simulink model "TRMSStateChart"  (R2020b)
settings: Solver=VariableStepAuto  StartTime=0.0  StopTime=inf  RelTol=1e-3
libraries: simulink x2
settings Model: EnablePacing=on  Creator=Ahmed Zaghloul  LastModifiedBy=Ahmed Zaghloul

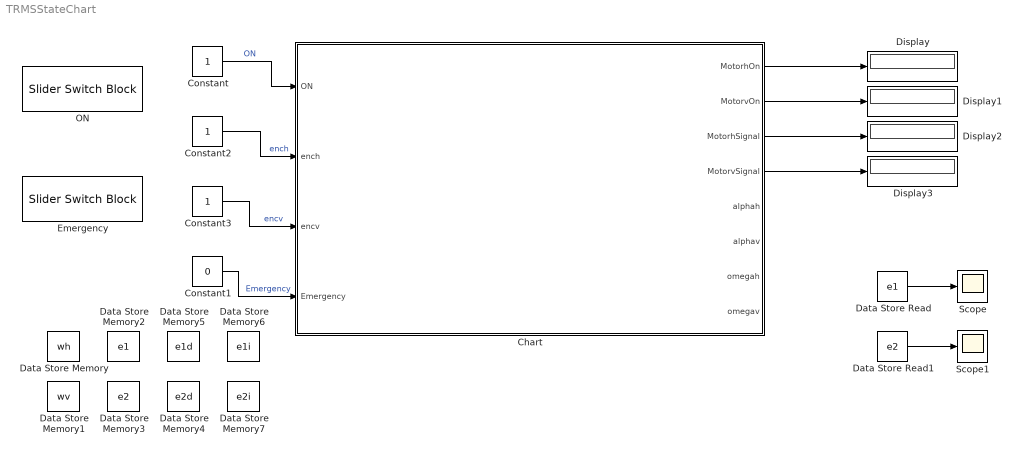
== system TRMSStateChart ==
  Chart : Stateflow chart  TreatAsAtomicUnit=on
  Constant : Constant
  Constant1 : Constant  Value=0
  Constant2 : Constant
  Constant3 : Constant
  Data Store Read : DataStoreRead  DataStoreName=e1
  Data Store Read1 : DataStoreRead  DataStoreName=e2
  Data Store Memory : DataStoreMemory  DataStoreName=wh  ReadBeforeWriteMsg=warning  WriteAfterWriteMsg=warning  WriteAfterReadMsg=warning  ShowAdditionalParam=off  OutDataTypeStr=double
  Data Store Memory1 : DataStoreMemory  DataStoreName=wv  ReadBeforeWriteMsg=warning  WriteAfterWriteMsg=warning  WriteAfterReadMsg=warning  ShowAdditionalParam=off  OutDataTypeStr=double
  Data Store Memory2 : DataStoreMemory  DataStoreName=e1  ReadBeforeWriteMsg=warning  WriteAfterWriteMsg=warning  WriteAfterReadMsg=warning  ShowAdditionalParam=off  OutDataTypeStr=double
  Data Store Memory3 : DataStoreMemory  DataStoreName=e2  ReadBeforeWriteMsg=warning  WriteAfterWriteMsg=warning  WriteAfterReadMsg=warning  ShowAdditionalParam=off  OutDataTypeStr=double
  Data Store Memory4 : DataStoreMemory  DataStoreName=e2d  ReadBeforeWriteMsg=warning  WriteAfterWriteMsg=warning  WriteAfterReadMsg=warning  ShowAdditionalParam=off  OutDataTypeStr=double
  Data Store Memory5 : DataStoreMemory  DataStoreName=e1d  ReadBeforeWriteMsg=warning  WriteAfterWriteMsg=warning  WriteAfterReadMsg=warning  ShowAdditionalParam=off  OutDataTypeStr=double
  Data Store Memory6 : DataStoreMemory  DataStoreName=e1i  ReadBeforeWriteMsg=warning  WriteAfterWriteMsg=warning  WriteAfterReadMsg=warning  ShowAdditionalParam=off  OutDataTypeStr=double
  Data Store Memory7 : DataStoreMemory  DataStoreName=e2i  ReadBeforeWriteMsg=warning  WriteAfterWriteMsg=warning  WriteAfterReadMsg=warning  ShowAdditionalParam=off  OutDataTypeStr=double
  Display{,1..3} (4 alike) : Display
  Emergency : SliderSwitchBlock
      settings: Values={{'Off', 'On'}, [0 1]}
  ON : SliderSwitchBlock
      settings: Values={{'Off', 'On'}, [0 1]}
  Scope : Scope
  Scope1 : Scope
  wires:
  Constant/1 -> Chart/1(ON)  "ON"
  Constant1/1 -> Chart/4(Emergency)  "Emergency"
  Chart/1(MotorhOn) -> Display/1
  Chart/2(MotorvOn) -> Display1/1
  Chart/3(MotorhSignal) -> Display2/1
  Chart/4(MotorvSignal) -> Display3/1
  Constant2/1 -> Chart/2(ench)  "ench"
  Constant3/1 -> Chart/3(encv)  "encv"
  Data Store Read/1 -> Scope/1
  Data Store Read1/1 -> Scope1/1

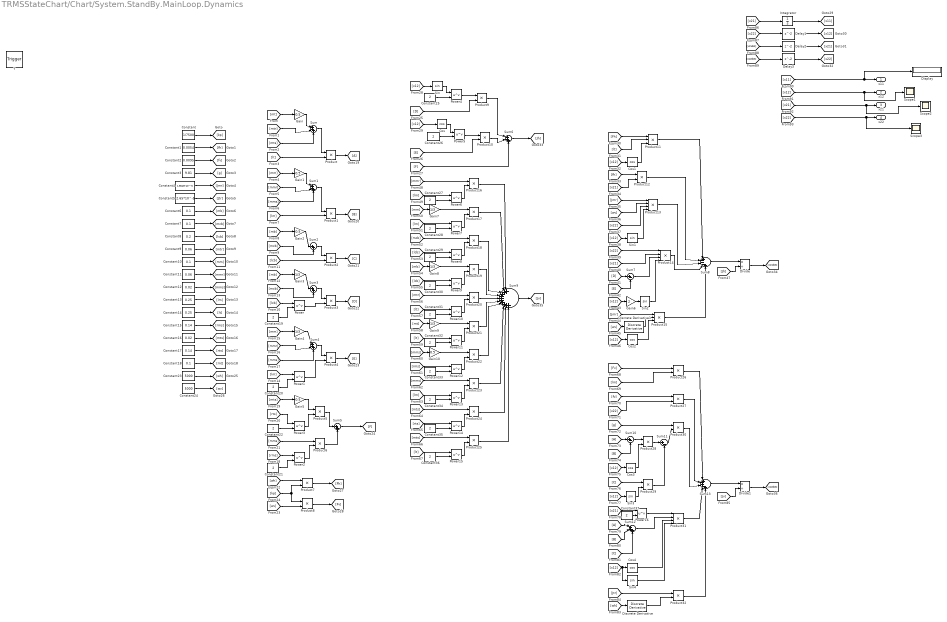
== system TRMSStateChart/Chart/System.StandBy.MainLoop.Dynamics ==
  f : TriggerPort  TriggerType=function-call  VariantControl=(inherit)  SampleTime=-1
      settings: CopyFcn=Stateflow.SLINSF.SimulinkMan.removeBlockPreDeleteFcn  PreDeleteFcn=Stateflow.SLINSF.SimulinkMan.unsafePredeleteFcn
  Constant : Constant  Value=1/7500
  Constant1 : Constant  Value=0.0054
  Constant{6..7,10,18} (4 alike) : Constant  Value=0.1
  Constant11 : Constant  Value=0.06
  Constant12 : Constant  Value=0.02
  Constant13 : Constant  Value=0.25
  Constant14 : Constant  Value=0.25
  Constant15 : Constant  Value=0.14
  Constant16 : Constant  Value=0.02
  Constant17 : Constant  Value=0.14
  Constant{19..22,25..37} (17 alike) : Constant  Value=2
  Constant2 : Constant  Value=0.0095
  Constant23 : Constant  Value=5000
  Constant24 : Constant  Value=5000
  Constant3 : Constant  Value=9.81
  Constant4 : Constant  Value=1.6543*10^-5
  Constant5 : Constant  Value=2.65*10^-5
  Constant8 : Constant  Value=0.2
  Constant9 : Constant  Value=0.06
  Cos{,1..4} (5 alike) : Trigonometry  Operator=cos
  Delay1 : Delay
  Delay2 : Delay
  Delay3 : Delay
  Discrete Derivative : simulink/Discrete/Discrete Derivative  gainval=1.0  ICPrevScaledInput=0.0  OutMin=[]  OutMax=[]  OutDataType=fixdt(1, 16)  OutScaling=2^-10  DoSatur=off
  Discrete Derivative1 : simulink/Discrete/Discrete Derivative  gainval=1.0  ICPrevScaledInput=0.0  OutMin=[]  OutMax=[]  OutDataType=fixdt(1, 16)  OutScaling=2^-10  DoSatur=off
  Display : Display
  Divide : Product  Inputs=*/
  Divide1 : Product  Inputs=*/
  Gain{,1..2,5,10} (5 alike) : Gain  Gain=0.5
  Gain{3..4,7..9} (5 alike) : Gain  Gain=1/3
  Gain6 : Gain  Gain=2
  Integrator : Integrator
  Power{,1..16} (17 alike) : Math  Operator=pow  SaturateOnIntegerOverflow=on
  Product{,1..10,12,16..30,32} (28 alike) : Product
  Product11 : Product  Inputs=3
  Product13 : Product  Inputs=4
  Product14 : Product  Inputs=4
  Product15 : Product  Inputs=3
  Product31 : Product  Inputs=4
  Scope1 : Scope
  Scope2 : Scope
  Scope3 : Scope
  Sin{,1..4} (5 alike) : Trigonometry
  Sum{,1,4,6,12} (5 alike) : Sum  Inputs=|+++
  Sum10 : Sum  Inputs=|+-
  Sum11 : Sum  Inputs=|+-
  Sum13 : Sum  Inputs=|+-+-+
  Sum2 : Sum  Inputs=|++
  Sum3 : Sum  Inputs=|++
  Sum5 : Sum  Inputs=|++
  Sum7 : Sum  Inputs=|+-
  Sum8 : Sum  Inputs=|+---+
  Sum9 : Sum  Inputs=|++++++++++
  x11 : Outport
  x12 : Outport  Port=2
  x21 : Outport  Port=3
  x22 : Outport  Port=4
  wires:
  Constant/1 -> [kp]
  Constant1/1 -> [fh]
  Constant2/1 -> [fv]
  Constant3/1 -> [g]
  Constant4/1 -> [Jmr]
  Constant5/1 -> [Jtr]
  Constant6/1 -> [mb]
  Constant7/1 -> [mcb]
  Constant8/1 -> [lcb]
  Constant9/1 -> [mtr]
  Constant10/1 -> [mm]
  Constant11/1 -> [mmr]
  Constant12/1 -> [mms]
  Constant13/1 -> [lm]
  Constant14/1 -> [lt]
  Constant15/1 -> [rms]
  Constant16/1 -> [mts]
  Constant17/1 -> [rts]
  [mt] -> Gain/1
  Constant18/1 -> [mt]
  Gain/1 -> Sum/1
  [mtr] -> Sum/2
  [mts] -> Sum/3
  [lt] -> Product/2
  Sum/1 -> Product/1
  Product/1 -> [A]
  Product1/1 -> [B]
  Sum1/1 -> Product1/1
  [lm] -> Product1/2
  [mms] -> Sum1/3
  [mmr] -> Sum1/2
  Gain1/1 -> Sum1/1
  [mm] -> Gain1/1
  Gain2/1 -> Sum2/1
  [lcb] -> Product2/2
  [mb] -> Gain2/1
  Product2/1 -> [C]
  [mcb] -> Sum2/2
  Sum2/1 -> Product2/1
  Sum3/1 -> Product3/1
  [mcb] -> Sum3/2
  Product3/1 -> [D]
  [mb] -> Gain3/1
  Gain3/1 -> Sum3/1
  [lcb] -> Power/1
  Constant19/1 -> Power/2
  Power/1 -> Product3/2
  Power1/1 -> Product4/2
  Constant20/1 -> Power1/2
  [lm] -> Power1/1
  Gain4/1 -> Sum4/1
  [mm] -> Gain4/1
  Product4/1 -> [E]
  [mmr] -> Sum4/2
  Sum4/1 -> Product4/1
  [mms] -> Sum4/3
  [rts] -> Power3/1
  Sum5/1 -> [F]
  [mts] -> Gain5/1
  Gain5/1 -> Product5/1
  [rms] -> Power2/1
  Constant21/1 -> Power2/2
  Constant22/1 -> Power3/2
  Power3/1 -> Product5/2
  Power2/1 -> Product6/2
  [mms] -> Product6/1
  Product5/1 -> Sum5/1
  Product6/1 -> Sum5/2
  Constant23/1 -> [wh]
  Constant24/1 -> [wv]
  [wh] -> Product7/1
  [kp] -> Product8/1, Product7/2
  [wv] -> Product8/2
  Product7/1 -> [Fh]
  Product8/1 -> [Fv]
  [x12] -> Sin/1
  Constant25/1 -> Power4/2
  Constant26/1 -> Power5/2
  Sin/1 -> Power4/1
  Power4/1 -> Product9/1
  [D] -> Product9/2
  [x12] -> Cos/1
  Cos/1 -> Power5/1
  Power5/1 -> Product10/1
  [E] -> Product10/2
  Product9/1 -> Sum6/1
  Product10/1 -> Sum6/2
  [F] -> Sum6/3
  Sum6/1 -> [Jh]
  [x12] -> Cos1/1
  [Fh] -> Product11/1
  [lt] -> Product11/2
  Cos1/1 -> Product11/3
  [fh] -> Product12/1
  [x21] -> Product12/2
  [x12] -> Sin1/1
  [Jmr] -> Product13/1
  [wv] -> Product13/2
  [x22] -> Product13/3
  Sin1/1 -> Product13/4
  [x12] -> Gain6/1
  Gain6/1 -> Sin2/1
  [x22] -> Product14/1
  [x21] -> Product14/2
  [D] -> Sum7/1
  [E] -> Sum7/2
  Sum7/1 -> Product14/3
  Sin2/1 -> Product14/4
  [x12] -> Cos2/1
  [Jmr] -> Product15/1
  Cos2/1 -> Product15/3
  Product11/1 -> Sum8/1
  Product12/1 -> Sum8/2
  Product13/1 -> Sum8/3
  Product14/1 -> Sum8/4
  Product15/1 -> Sum8/5
  Sum8/1 -> Divide/1
  [Jh] -> Divide/2
  Divide/1 -> [x21dot]
  [lm] -> Power6/1
  Constant27/1 -> Power6/2
  Power6/1 -> Product16/2
  [mmr] -> Product16/1
  [mm] -> Gain7/1
  Constant28/1 -> Power7/2
  [lm] -> Power7/1
  Gain7/1 -> Product17/1
  Power7/1 -> Product17/2
  [lcb] -> Power8/1
  Constant29/1 -> Power8/2
  [mcb] -> Product18/1
  Power8/1 -> Product18/2
  [mb] -> Gain8/1
  Constant30/1 -> Power9/2
  [lcb] -> Power9/1
  Gain8/1 -> Product19/1
  Power9/1 -> Product19/2
  Constant31/1 -> Power10/2
  [lt] -> Power10/1
  [mtr] -> Product20/1
  Power10/1 -> Product20/2
  [mt] -> Gain9/1
  Constant32/1 -> Power11/2
  [lt] -> Power11/1
  Gain9/1 -> Product21/1
  Power11/1 -> Product21/2
  [mms] -> Gain10/1
  Constant33/1 -> Power12/2
  [rms] -> Power12/1
  Gain10/1 -> Product22/1
  Power12/1 -> Product22/2
  Constant34/1 -> Power13/2
  [lm] -> Power13/1
  [mms] -> Product23/1
  Power13/1 -> Product23/2
  [lt] -> Power15/1
  [rts] -> Power14/1
  Constant36/1 -> Power15/2
  Constant35/1 -> Power14/2
  [mts] -> Product24/1
  Power14/1 -> Product24/2
  [mts] -> Product25/1
  Power15/1 -> Product25/2
  Product16/1 -> Sum9/1
  Product17/1 -> Sum9/2
  Product18/1 -> Sum9/3
  Product19/1 -> Sum9/4
  Product20/1 -> Sum9/5
  Product21/1 -> Sum9/6
  Product22/1 -> Sum9/7
  Product23/1 -> Sum9/8
  Product24/1 -> Sum9/9
  Product25/1 -> Sum9/10
  Sum9/1 -> [Jv]
  [Fv] -> Product26/1
  [lm] -> Product26/2
  [fv] -> Product27/1
  [x22] -> Product27/2
  [A] -> Sum10/1
  [B] -> Sum10/2
  [x12] -> Cos3/1
  Sum10/1 -> Product28/1
  Cos3/1 -> Product28/2
  [x12] -> Sin3/1
  Sin3/1 -> Product29/2
  [C] -> Product29/1
  Product28/1 -> Sum11/1
  Product29/1 -> Sum11/2
  [g] -> Product30/1
  Sum11/1 -> Product30/2
  Constant37/1 -> Power16/2
  [x21] -> Power16/1
  [A] -> Sum12/1
  [B] -> Sum12/2
  [C] -> Sum12/3
  [x12] -> Sin4/1, Cos4/1
  Power16/1 -> Product31/1
  Sum12/1 -> Product31/2
  Cos4/1 -> Product31/3
  Sin4/1 -> Product31/4
  [Jtr] -> Product32/1
  [wh] -> Discrete Derivative/1
  Product26/1 -> Sum13/1
  Product27/1 -> Sum13/2
  Product30/1 -> Sum13/3
  Product31/1 -> Sum13/4
  Product32/1 -> Sum13/5
  Sum13/1 -> Divide1/1
  [Jv] -> Divide1/2
  Divide1/1 -> [x22dot]
  Integrator/1 -> [x11]
  [x21] -> Integrator/1
  [x22] -> Delay1/1
  [x21dot] -> Delay2/1
  [x22dot] -> Delay3/1
  [x11] -> Display/1, x11/1
  [x12] -> Scope1/1, x12/1
  [x21] -> Scope2/1, x21/1
  [x22] -> Scope3/1, x22/1
  Delay1/1 -> [x12]
  Delay2/1 -> [x21]
  Delay3/1 -> [x22]
  Discrete Derivative/1 -> Product32/2
  [wv] -> Discrete Derivative1/1
  Discrete Derivative1/1 -> Product15/2

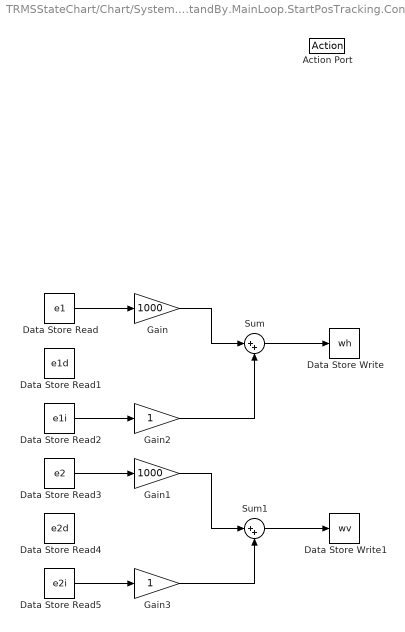
== system TRMSStateChart/Chart/System.StandBy.MainLoop.StartPosTracking.Controller ==
  Action Port : ActionPort
      settings: CopyFcn=Stateflow.SLINSF.SimulinkMan.removeBlockPreDeleteFcn  PreDeleteFcn=Stateflow.SLINSF.SimulinkMan.unsafePredeleteFcn
  Data Store Read : DataStoreRead  DataStoreName=e1
  Data Store Read1 : DataStoreRead  DataStoreName=e1d
  Data Store Read2 : DataStoreRead  DataStoreName=e1i
  Data Store Read3 : DataStoreRead  DataStoreName=e2
  Data Store Read4 : DataStoreRead  DataStoreName=e2d
  Data Store Read5 : DataStoreRead  DataStoreName=e2i
  Data Store Write : DataStoreWrite  DataStoreName=wh
  Data Store Write1 : DataStoreWrite  DataStoreName=wv
  Gain : Gain  Gain=1000
  Gain1 : Gain  Gain=1000
  Gain2 : Gain
  Gain3 : Gain
  Sum : Sum  Inputs=|++
  Sum1 : Sum  Inputs=|++
  wires:
  Data Store Read/1 -> Gain/1
  Data Store Read3/1 -> Gain1/1
  Data Store Read2/1 -> Gain2/1
  Data Store Read5/1 -> Gain3/1
  Gain/1 -> Sum/1
  Gain2/1 -> Sum/2
  Gain1/1 -> Sum1/1
  Gain3/1 -> Sum1/2
  Sum/1 -> Data Store Write/1
  Sum1/1 -> Data Store Write1/1

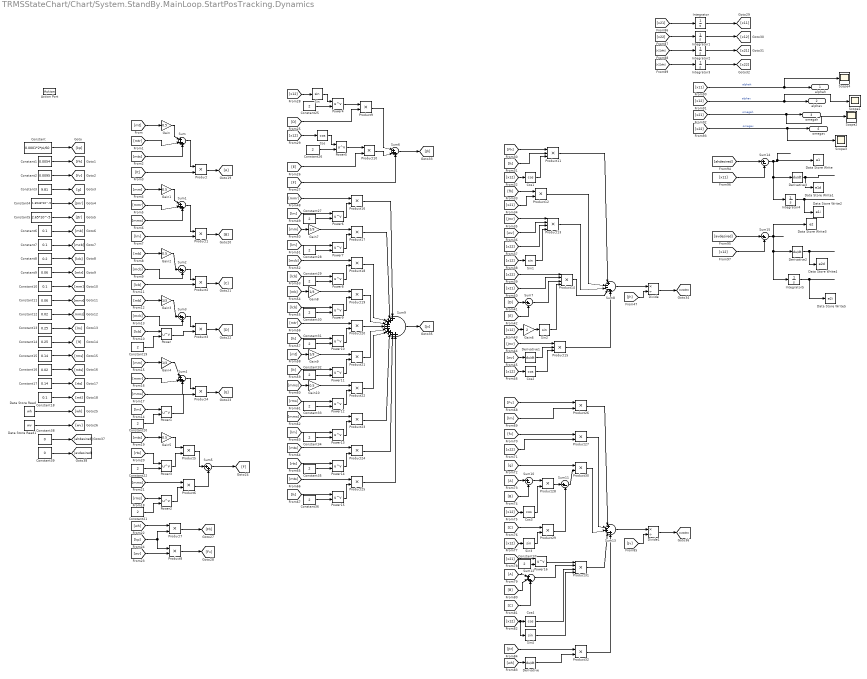
== system TRMSStateChart/Chart/System.StandBy.MainLoop.StartPosTracking.Dynamics ==
  Action Port : ActionPort
      settings: CopyFcn=Stateflow.SLINSF.SimulinkMan.removeBlockPreDeleteFcn  PreDeleteFcn=Stateflow.SLINSF.SimulinkMan.unsafePredeleteFcn
  Constant : Constant  Value=0.0001*2*pi/60
  Constant1 : Constant  Value=0.0054
  Constant{6..7,10,18} (4 alike) : Constant  Value=0.1
  Constant11 : Constant  Value=0.06
  Constant12 : Constant  Value=0.02
  Constant13 : Constant  Value=0.25
  Constant14 : Constant  Value=0.25
  Constant15 : Constant  Value=0.14
  Constant16 : Constant  Value=0.02
  Constant17 : Constant  Value=0.14
  Constant{19..22,25..37} (17 alike) : Constant  Value=2
  Constant2 : Constant  Value=0.0095
  Constant3 : Constant  Value=9.81
  Constant38 : Constant  Value=0
  Constant39 : Constant  Value=0
  Constant4 : Constant  Value=1.6543*10^-5
  Constant5 : Constant  Value=2.65*10^-5
  Constant8 : Constant  Value=0.2
  Constant9 : Constant  Value=0.06
  Cos{,1..4} (5 alike) : Trigonometry  Operator=cos
  Data Store Read : DataStoreRead  DataStoreName=wh
  Data Store Read1 : DataStoreRead  DataStoreName=wv
  Data Store Write : DataStoreWrite  DataStoreName=e1
  Data Store Write1 : DataStoreWrite  DataStoreName=e1d
  Data Store Write2 : DataStoreWrite  DataStoreName=e1i
  Data Store Write3 : DataStoreWrite  DataStoreName=e2
  Data Store Write4 : DataStoreWrite  DataStoreName=e2d
  Data Store Write5 : DataStoreWrite  DataStoreName=e2i
  Derivative{,1..3} (4 alike) : Derivative
  Divide : Product  Inputs=*/
  Divide1 : Product  Inputs=*/
  Gain{,1..2,5,10} (5 alike) : Gain  Gain=0.5
  Gain{3..4,7..9} (5 alike) : Gain  Gain=1/3
  Gain6 : Gain  Gain=2
  Integrator : Integrator  InitialCondition=0.1  WrapState=on  ContinuousStateAttributes='alphah'
  Integrator1 : Integrator  InitialCondition=0.1  WrapState=on  ContinuousStateAttributes='alphav'
  Integrator{2..5} (4 alike) : Integrator  ContinuousStateAttributes='omegah'
  Power{,1..16} (17 alike) : Math  Operator=pow  SaturateOnIntegerOverflow=on
  Product{,1..10,12,16..30,32} (28 alike) : Product
  Product11 : Product  Inputs=3
  Product13 : Product  Inputs=4
  Product14 : Product  Inputs=4
  Product15 : Product  Inputs=3
  Product31 : Product  Inputs=4
  Scope{1..4} (4 alike) : Scope
  Sin{,1..4} (5 alike) : Trigonometry
  Sum{,1,4,6,12} (5 alike) : Sum  Inputs=|+++
  Sum{7,10..11,14..15} (5 alike) : Sum  Inputs=|+-
  Sum13 : Sum  Inputs=|+-+-+
  Sum2 : Sum  Inputs=|++
  Sum3 : Sum  Inputs=|++
  Sum5 : Sum  Inputs=|++
  Sum8 : Sum  Inputs=|+---+
  Sum9 : Sum  Inputs=|++++++++++
  alphah : Outport
  alphav : Outport  Port=2
  omegah : Outport  Port=3
  omegav : Outport  Port=4
  wires:
  [x21] -> Integrator/1
  Constant3/1 -> [g]
  [mcb] -> Product18/1
  [F] -> Sum6/3
  [mm] -> Gain4/1
  Gain3/1 -> Sum3/1
  [C] -> Product29/1
  [fh] -> Product12/1
  [wh] -> Product7/1
  [x21] -> Power16/1
  [mb] -> Gain2/1
  Constant7/1 -> [mcb]
  [lm] -> Power6/1
  [x12] -> Sin4/1, Cos4/1
  Constant37/1 -> Power16/2
  Constant36/1 -> Power15/2
  [Jtr] -> Product32/1
  Product15/1 -> Sum8/5
  [rts] -> Power14/1
  Sin3/1 -> Product29/2
  Gain2/1 -> Sum2/1
  Constant5/1 -> [Jtr]
  [E] -> Product10/2
  Constant8/1 -> [lcb]
  Product2/1 -> [C]
  Gain10/1 -> Product22/1
  Product21/1 -> Sum9/6
  Sum10/1 -> Product28/1
  Product5/1 -> Sum5/1
  [x12] -> Cos3/1
  Constant21/1 -> Power2/2
  Sum/1 -> Product/1
  [lcb] -> Power9/1
  Sum9/1 -> [Jv]
  Product24/1 -> Sum9/9
  Product18/1 -> Sum9/3
  [x12] -> Cos/1
  Sum1/1 -> Product1/1
  [x22] -> Product27/2
  Divide/1 -> [x21dot]
  Constant34/1 -> Power13/2
  Power11/1 -> Product21/2
  [Jmr] -> Product15/1
  [mms] -> Product23/1
  Gain4/1 -> Sum4/1
  [wv] -> Product13/2
  Gain9/1 -> Product21/1
  [rms] -> Power12/1
  Power/1 -> Product3/2
  [mms] -> Gain10/1
  Constant33/1 -> Power12/2
  Constant28/1 -> Power7/2
  [mts] -> Product24/1
  [lt] -> Power15/1
  Gain8/1 -> Product19/1
  Power8/1 -> Product18/2
  [lt] -> Power11/1
  [lt] -> Power10/1
  Constant31/1 -> Power10/2
  Product7/1 -> [Fh]
  Constant35/1 -> Power14/2
  Constant32/1 -> Power11/2
  [mt] -> Gain/1
  Sum5/1 -> [F]
  [mtr] -> Product20/1
  Power9/1 -> Product19/2
  Constant30/1 -> Power9/2
  Sum8/1 -> Divide/1
  [Jh] -> Divide/2
  [lm] -> Power7/1
  Constant20/1 -> Power1/2
  [x21] -> Product14/2
  [mmr] -> Product16/1
  Constant27/1 -> Power6/2
  Gain7/1 -> Product17/1
  Product9/1 -> Sum6/1
  Product13/1 -> Sum8/3
  [lcb] -> Power8/1
  [x12] -> Cos2/1
  [mts] -> Gain5/1
  Cos2/1 -> Product15/3
  Power7/1 -> Product17/2
  Product1/1 -> [B]
  Cos/1 -> Power5/1
  [E] -> Sum7/2
  Product27/1 -> Sum13/2
  Sin2/1 -> Product14/4
  [x22] -> Product14/1
  Constant2/1 -> [fv]
  [x12] -> Gain6/1
  Sum11/1 -> Product30/2
  Constant15/1 -> [rms]
  Constant17/1 -> [rts]
  Gain6/1 -> Sin2/1
  Sum7/1 -> Product14/3
  Product6/1 -> Sum5/2
  Gain/1 -> Sum/1
  [C] -> Sum12/3
  Sin/1 -> Power4/1
  Constant26/1 -> Power5/2
  Product22/1 -> Sum9/7
  [x12] -> Sin/1
  Cos3/1 -> Product28/2
  [D] -> Product9/2
  [Fh] -> Product11/1
  Product29/1 -> Sum11/2
  Product8/1 -> [Fv]
  Sum6/1 -> [Jh]
  [lm] -> Product1/2
  Product10/1 -> Sum6/2
  [wv] -> Product8/2
  Constant25/1 -> Power4/2
  [x12] -> Cos1/1
  Constant19/1 -> Power/2
  [x21] -> Product12/2
  Power5/1 -> Product10/1
  [kp] -> Product8/1, Product7/2
  Power13/1 -> Product23/2
  Product4/1 -> [E]
  [mm] -> Gain7/1
  [lcb] -> Product2/2
  Constant29/1 -> Power8/2
  Power3/1 -> Product5/2
  [mmr] -> Sum4/2
  [lm] -> Power1/1
  Constant1/1 -> [fh]
  [mm] -> Gain1/1
  Sin1/1 -> Product13/4
  [rms] -> Power2/1
  [mcb] -> Sum3/2
  [mms] -> Product6/1
  Product17/1 -> Sum9/2
  [mb] -> Gain3/1
  [lm] -> Product26/2
  [mts] -> Sum/3
  [lcb] -> Power/1
  Constant9/1 -> [mtr]
  [mmr] -> Sum1/2
  Constant14/1 -> [lt]
  Product/1 -> [A]
  Constant13/1 -> [lm]
  [lt] -> Product/2
  Gain1/1 -> Sum1/1
  Constant10/1 -> [mm]
  [mms] -> Sum1/3
  [mtr] -> Sum/2
  Constant18/1 -> [mt]
  Constant11/1 -> [mmr]
  Cos4/1 -> Product31/3
  Constant/1 -> [kp]
  Derivative/1 -> Product32/2
  [x22] -> Integrator1/1
  Power15/1 -> Product25/2
  [x12] -> Sin1/1
  Product14/1 -> Sum8/4
  [x12] -> Sin3/1
  Power6/1 -> Product16/2
  Product11/1 -> Sum8/1
  [x22] -> omegav/1, Scope3/1  "omegav"
  Product23/1 -> Sum9/8
  Sum4/1 -> Product4/1
  Constant22/1 -> Power3/2
  Product30/1 -> Sum13/3
  [x21] -> omegah/1, Scope2/1  "omegah"
  [lt] -> Product11/2
  Product3/1 -> [D]
  Integrator3/1 -> [x22]
  [lm] -> Power13/1
  [wv] -> Derivative1/1
  [mms] -> Sum4/3
  [x11] -> Scope4/1, alphah/1  "alphah"
  Product12/1 -> Sum8/2
  Sum2/1 -> Product2/1
  [x22] -> Product13/3
  Product25/1 -> Sum9/10
  Power10/1 -> Product20/2
  Sum12/1 -> Product31/2
  [mt] -> Gain9/1
  [x12] -> alphav/1, Scope1/1  "alphav"
  [D] -> Sum7/1
  [wh] -> Derivative/1
  Product26/1 -> Sum13/1
  Product16/1 -> Sum9/1
  Product28/1 -> Sum11/1
  Derivative1/1 -> Product15/2
  Constant6/1 -> [mb]
  [B] -> Sum12/2
  Sum3/1 -> Product3/1
  Product20/1 -> Sum9/5
  Product32/1 -> Sum13/5
  [x21dot] -> Integrator2/1
  [Fv] -> Product26/1
  Power2/1 -> Product6/2
  [fv] -> Product27/1
  [rts] -> Power3/1
  [mcb] -> Sum2/2
  [x22dot] -> Integrator3/1
  Divide1/1 -> [x22dot]
  Product19/1 -> Sum9/4
  [mb] -> Gain8/1
  Constant12/1 -> [mms]
  Sum13/1 -> Divide1/1
  Power16/1 -> Product31/1
  [A] -> Sum12/1
  Power1/1 -> Product4/2
  Constant16/1 -> [mts]
  [mts] -> Product25/1
  Power4/1 -> Product9/1
  [A] -> Sum10/1
  Sin4/1 -> Product31/4
  Constant4/1 -> [Jmr]
  Power12/1 -> Product22/2
  [Jmr] -> Product13/1
  [B] -> Sum10/2
  Integrator2/1 -> [x21]
  Gain5/1 -> Product5/1
  [Jv] -> Divide1/2
  Product31/1 -> Sum13/4
  Cos1/1 -> Product11/3
  [g] -> Product30/1
  Power14/1 -> Product24/2
  Constant38/1 -> [ahdesired]
  Constant39/1 -> [avdesired]
  [ahdesired] -> Sum14/1
  [x11] -> Sum14/2
  [avdesired] -> Sum15/1
  [x12] -> Sum15/2
  Sum14/1 -> Integrator4/1, Derivative3/1, Data Store Write/1
  Derivative3/1 -> Data Store Write1/1
  Derivative2/1 -> Data Store Write4/1
  Integrator4/1 -> Data Store Write2/1
  Integrator5/1 -> Data Store Write5/1
  Sum15/1 -> Data Store Write3/1, Integrator5/1, Derivative2/1
  Integrator/1 -> [x11]
  Integrator1/1 -> [x12]
  Data Store Read/1 -> [wh]
  Data Store Read1/1 -> [wv]

== stateflow chart TRMSStateChart/Chart ==
  state System
    state StandBy
      entry:
      MotorhOn = 1
      MotorvOn = 1
      motorcalibration = 0
      sensorcalibration = 0
      state MainLoop
        entry:
        alphah = 0
        alphav = 0
        omegah = 0
        omegav = 0
        e1 = 0
        e1d = 0
        e1i = 0
        e2 = 0
        e2d = 0
        e2i = 0
        state StartPosTracking
          state Controller [parallel]
            settings: executionOrder=1
          state Dynamics [parallel]
            settings: executionOrder=2
        state Controller [commented out]
          during:
          wh = kp*e1 + ki*e1i + kd*e1d
          wv = kp*e2 + ki*e2i + kd*e2d
        state [x11,x12,x21,x22] = Dynamics [function] [commented out]
        (default) -> StartPosTracking
      state Calibration
        state MotorCalibration [parallel]
          settings: executionOrder=1
          state High
            entry:MotorhSignal = 2000
            MotorvSignal = 2000
          state Low
            entry:MotorhSignal = 1000
            MotorvSignal = 1000
          state FinishCalibrationMotor
            entry:
            wv = 0
            wh = 0
            motorcalibration = 1
          (default) -> High
          High -> Low : after(2,sec)
          Low -> FinishCalibrationMotor
        state SensorCalibration [parallel]
          settings: executionOrder=2
          state ReadData
            entry:
            zeroPosh = ench
            zeroPosv = encv
          state FinishCalibrationSensor
            entry:
            sensorcalibration = 1
          (default) -> ReadData
          ReadData -> FinishCalibrationSensor : after(2,sec)
      (default) -> Calibration
      Calibration -> MainLoop : [motorcalibration == 1 && sensorcalibration == 1]
    state OFF
      entry:
      MotorhOn = 0
      MotorvOn = 0
    state Emergency
      entry:
      MotorhOn = 0
      MotorvOn = 0
    (default) -> OFF
    StandBy -> OFF [order 1] : [ON == 0]
    OFF -> StandBy : [ON == 1]
    StandBy -> Emergency [order 2] : [Emergency == 1]
    Emergency -> StandBy : [Emergency == 0]
  (default) -> System
  data: sf_internal_action_state_placeholder_data local double size=1 =0; sf_internal_action_state_placeholder_data local double size=1 =0; x11 function_output double size=1; x12 function_output double size=1; x21 function_output double size=1; x22 function_output double size=1; ON input size=1; ench input; encv input; Emergency input; MotorhOn output; MotorvOn output; MotorhSignal output; MotorvSignal output; zeroPosh local; zeroPosv local; motorcalibration local; sensorcalibration local; Dynamics local; alphah output; alphav output; omegah output; omegav output; kp constant double =5000; kd constant double =0; ki constant double =0.01; wh data_store_memory; wv data_store_memory; e1 data_store_memory; e1d data_store_memory; e1i data_store_memory; e2 data_store_memory; e2d data_store_memory; e2i data_store_memory
